simulink model "boat_dynamics_model"  (R2025a)
settings: Solver=ode4  StartTime=0.0  StopTime=10  FixedStep=Ts_sim  RelTol=1e-3
values from neighbouring files (symbols this model uses):
  ctrl_params = boat_controller_parameters()    [setup_MDL.m]
  plant_params = boat_model_parameters_3dof()    [setup_MDL.m]
  u0 = u0(:)    [find_A_B_LQR.m]    (also in find_equilibrium_3dof.m = zeros(5,1); setup_MDL.m = trim.u0; tmp_continuous_controller.mat = [1.84671066471 1.84671066471 1.93397466068 0 3]; tmp_discrete_controller.mat = [1.84671066471 1.84671066471 1.93397466068 0 3])
  x0 = x0(:)    [find_A_B_LQR.m]    (also in find_equilibrium_3dof.m = zeros(11,1); setup_MDL.m = trim.x0; tmp_continuous_controller.mat = [-0.1 0 0 0 0 0 0 0 1.84671066471 1.84671066471 1.9339746606; tmp_discrete_controller.mat = [-0.1 0 0 0 0 0 0 0 1.84671066471 1.84671066471 1.9339746606)
undefined symbols (not defined in the file or in its folder): Ts_sim
libraries: simulink_extras x2, sim3dlib x2, rllib x1
settings Model: Creator=brzan  LastModifiedBy=brzan

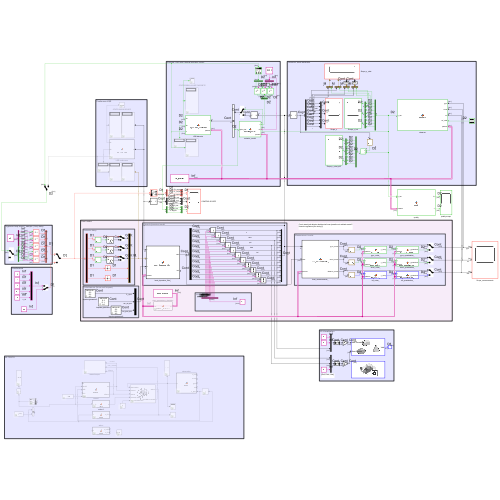
[thumbnail: Simulink's stored preview of the top-level diagram]
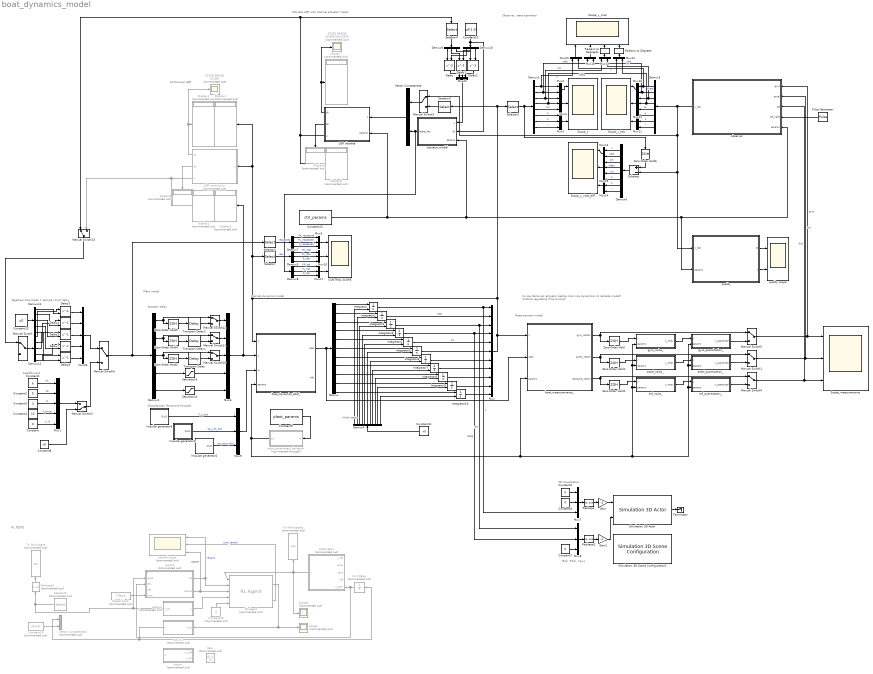
== system boat_dynamics_model ==
  note: Plant model
  note: Actuator delay
  note: Algebraic loop break 1 sample (1ms) delay
  note: RL TESTS
  note: Observer, state estimator
  note: Co sie stanie jak aktuator bedzie mial inna dynamike niz zaklada model?
      | Uczenie regulatora (fine tuning?)
  note: Discrete LQR with Internal actuator model
  note: Continuous LQR
  note: Feedforward
  note: Measurement model
  note: Internal dynamics model
  note: Initial state
  note: Disturbances (force and forques)
  note: 3D Visualization
  note: [Roll, Pitch, Yaw]
  CONTROL SCOPE : Scope  NumInputPorts=3
      settings: ActiveDisplayYMinimum=1.6100937743534502  ActiveDisplayYMaximum=2.3589425832417694  DataLoggingVariableName=ScopeAction
  Constant{,5..7} (4 alike) : Constant  Value=0
  Constant1 : Constant  Value=6
  Constant10 : Constant  Value=u0(1:3)  VectorParams1D=off
  Constant11 : Constant  Value=x0  VectorParams1D=off
  Constant12 : Constant  Value=u0  VectorParams1D=off
  Constant13 : Constant  Value=ctrl_params  VectorParams1D=off  OutDataTypeStr=Bus: ctrl_params_bus
  Constant14 : Constant  Commented=on  Value=u0(4:5)  VectorParams1D=off
  Constant15 : Constant  Commented=on  Value=0
  Constant2 : Constant  Value=6
  Constant3 : Constant  Value=3
  Constant4 : Constant  Value=10
  Constant8 : Constant  Value=u0
  Constant9 : Constant  Value=plant_params  VectorParams1D=off  OutDataTypeStr=Bus: plant_params_bus
  Delay : Delay  DelayLength=3  InitialConditionSource=Input port  SampleTime=ctrl_params.Ts
      settings: InputPortMap=u0,p4
  Delay1 : Delay  DelayLength=3  InitialConditionSource=Input port  SampleTime=ctrl_params.Ts
      settings: InputPortMap=u0,p4
  Delay2 : Delay  DelayLength=3  InitialConditionSource=Input port  SampleTime=ctrl_params.Ts
      settings: InputPortMap=u0,p4
  Delay{3..5,7..8} (5 alike) : Delay  DelayLength=1  InitialConditionSource=Input port  SampleTime=Ts_sim
      settings: InputPortMap=u0,p4
  Demux : Demux  Outputs=11
  Demux1 : Demux  Outputs=8
  Demux{3,7..10} (5 alike) : Demux  Outputs=3
  Demux11 : Demux  Outputs=5
  Demux12 : Demux  Outputs=5
  Demux2 : Demux  Outputs=5
  Demux4 : Demux  Outputs=11
  Demux5 : Demux  Outputs=8
  Demux6 : Demux  Outputs=8
  Digital Clock : DigitalClock  Commented=on  SampleTime=0.01
  Display{1..8} (8 alike) : Display  Commented=on
  Gain : Gain  Gain=-1
  Gain1 : Gain  Gain=-1
  Impulse generator1 : Subsystem  mask{start=2, duration=.1, amplitude=0}
      mask prompts: start "Start time"; duration "Duration time"; amplitude "Impulse amplitude"
      mask Display:
      | disp([ ...
      |     "IMPULSE"; ...
      |     'S ', ...
      |     num2str(get_param(gcb, 'start')); ...
      |     'D ', ...
      |     num2str(get_param(gcb, "duration")); ...
      |     'A ', ...
      |     num2str(get_param(gcb, "amplitude")) ...
      | ]);
  Impulse generator2 : Subsystem  mask{start=2, duration=5, amplitude=0}
      mask prompts: start "Start time"; duration "Duration time"; amplitude "Impulse amplitude"
      mask Display:
      | disp([ ...
      |     "IMPULSE"; ...
      |     'S ', ...
      |     num2str(get_param(gcb, 'start')); ...
      |     'D ', ...
      |     num2str(get_param(gcb, "duration")); ...
      |     'A ', ...
      |     num2str(get_param(gcb, "amplitude")) ...
      | ]);
  Impulse generator3 : Subsystem  mask{start=0, duration=2, amplitude=0}
      mask prompts: start "Start time"; duration "Duration time"; amplitude "Impulse amplitude"
      mask Display:
      | disp([ ...
      |     "IMPULSE"; ...
      |     'S ', ...
      |     num2str(get_param(gcb, 'start')); ...
      |     'D ', ...
      |     num2str(get_param(gcb, "duration")); ...
      |     'A ', ...
      |     num2str(get_param(gcb, "amplitude")) ...
      | ]);
  Integrator : Integrator  InitialConditionSource=external  InitialCondition=-0.11
  Integrator{1,3..10} (9 alike) : Integrator  InitialConditionSource=external
  Integrator2 : Integrator  InitialConditionSource=external  InitialCondition=deg2rad(3)
  LQR continuous : MATLAB Function  Commented=on  TreatAsAtomicUnit=on
  LQR discrete : MATLAB Function  TreatAsAtomicUnit=on  SystemSampleTime=ctrl_params.Ts
  Manual Switch{,1,3..6,10..13} (10 alike) : ManualSwitch
  Manual Switch2 : ManualSwitch  CurrentSetting=0
  Mux : Mux  Inputs=11
  Mux1 : Mux  Inputs=5
  Mux{2,10,13,18..21} (7 alike) : Mux  Inputs=2
  Mux{3..5,7..9,11..12,14..17,22} (13 alike) : Mux  Inputs=3
  Mux23 : Mux  Inputs=5
  Mux6 : Mux  Inputs=5
  Pulse Generator : DiscretePulseGenerator  Period=10  SampleTime=ctrl_params.Ts
  RL Agent : rllib/RL Agent  Commented=on  Agent=agentObj  ExternalActionAsInput=on  ProvideLastAction=off  ProvideCumRwd=on  TreatAsDirectFeedthrough=on  UseStrictObservationDataTypes=off
  Radians to Degrees : simulink_extras/Transformations/Radians to Degrees
  Radians to Degrees1 : simulink_extras/Transformations/Radians to Degrees
  Reshape : Reshape  OutputDimensionality=Row vector (2-D)
  Reshape1 : Reshape  OutputDimensionality=Row vector (2-D)
  Reshape2 : Reshape  Commented=on
  STATE ERROR SCOPE : Scope  Commented=on
      settings: ActiveDisplayYMinimum=-0.17004569092279864  ActiveDisplayYMaximum=0.25579071640803624  DataLoggingVariableName=ScopeData3
  STATE ERROR SCOPE DISCRETE : Scope  Commented=on
      settings: ActiveDisplayYMinimum=-0.17004569092279864  ActiveDisplayYMaximum=0.25579071640803624  DataLoggingVariableName=ScopeData6
  Saturation3 : Saturate  UpperLimit=5  LowerLimit=0
  Saturation4 : Saturate  UpperLimit=5  LowerLimit=0
  Scope : Scope  Commented=on
      settings: ActiveDisplayYMinimum=-2.4199088465030929  ActiveDisplayYMaximum=1.3794615097714347  DataLoggingVariableName=ScopeData2
  Scope1 : Scope  Commented=on
      settings: ActiveDisplayYMinimum=0.99404961030066707  ActiveDisplayYMaximum=1.0007752200523612  DataLoggingVariableName=ScopeData4
  Scope_measurements : Scope  NumInputPorts=3
      settings: ActiveDisplayYMinimum=-1.41006075  ActiveDisplayYMaximum=1.1051827499999998
  Scope_x : Scope  NumInputPorts=3
      settings: ActiveDisplayYMinimum=-0.11336426588314241  ActiveDisplayYMaximum=0.018631710839364757
  Scope_x_hat : Scope  NumInputPorts=3
      settings: ActiveDisplayYMinimum=-0.16104234357264974  ActiveDisplayYMaximum=0.14683807575538765  DataLoggingVariableName=ScopeObservation
  Scope_x_xhat : Scope  NumInputPorts=4
      settings: ActiveDisplayYMinimum=-0.24045599939750117  ActiveDisplayYMaximum=0.052378489407279127  DataLoggingVariableName=ScopeData7
  Scope_x_xhat_diff : Scope  NumInputPorts=3
      settings: ActiveDisplayYMinimum=-0.10989376677955481  ActiveDisplayYMaximum=0.074956658726200817  DataLoggingVariableName=ScopeData5
  Selector : Selector  InputPortWidth=11  IndexOptions=Index vector (dialog)  Indices=[9 10 11]  OutputSizes=1
  Selector1 : Selector  InputPortWidth=5  IndexOptions=Index vector (dialog)  Indices=[1 2 3]  OutputSizes=1
  Selector2 : Selector  InputPortWidth=11  IndexOptions=Index vector (dialog)  Indices=[1 2 3 4 5 6 7 8]  OutputSizes=1
  Selector3 : Selector  InputPortWidth=11  IndexOptions=Index vector (dialog)  Indices=[1 2 3 4 5 6 7 8]  OutputSizes=1
  Selector4 : Selector  InputPortWidth=5  IndexOptions=Index vector (dialog)  Indices=[1 2 3]  OutputSizes=1
  Selector5 : Selector  Commented=on  InputPortWidth=5  IndexOptions=Index vector (dialog)  Indices=[1 2 3]  OutputSizes=1
  Simulation 3D Actor : sim3dlib/Simulation 3D Actor  Priority=1  ActorName=Boat  ParentName=Scene Origin  Operation=Create at setup  InitScriptText=|  SampleTime=-1  Translation=[0 0 0]  Rotation=[0 0 0]  Scale=[1 1 1]/1000  InputsText=Boat.Translation Boat.Rotation  aMode=5  ActorTag=Boat  ActorType=Sim3dActor  ID=C
      | % Reserved keywords:
      | % - Actor : handle to this actor object
      | % - World : handle to the world object
      | 
      | % Examples:
      | 
      | % Create a primitive geometry (optional)
      | % createShape(Actor, 'box', [1 1 1]);
      | 
      | % Initialize values (optional)
      | % Actor.Physics = true;
      | % Actor.Color = [1 0 0];
  Simulation 3D Scene Configuration1 : sim3dlib/Simulation 3D Scene Configuration  Priority=0  ProjectFormat=Default Scenes  SceneDesc=Open surface  ProjectName=C:\Program Files\MATLAB\R2025a\toolbox\shared\sim3d_projects\automotive_project_windows\UE\WindowsNoEditor\VehicleSimulation.exe  ScenePath=/Game/Maps/HwStrght  EnableOpenDRIVE=off  vehTagList={'Boat';'Custom';'Scene Origin'}  vehTag=Boat  AttachedCameraRelativeTranslation=[-4 -3 1]*1000*0.25  FreeCameraDefaultInitialTranslation=[-6, 0, 2]  AttachedCameraRelativeRotation=[0 -10 40]  FreeCameraDefaultInitialRotation=[0, -15, 0]  ViewpointName=Custom  FreeCameraInitialTranslation=[-5 0 1]  ViewpointTranslation=[0 0 0]  FreeCameraInitialRotation=[0 0 0]  ViewpointRotation=[0 0 0]  OpVisEn=off  Ts=.05  EnableWindow=on  EnableRemoteAccess=off  EnableWeather=off  SunAzimuth=90  SunAltitude=40.0  EnableGeospatialSun=off  Latitude=0  Longitude=0  Date=2023-01-01  Time=10:30:00  GeoTimeZone=-5.0  SunDaylightSaving=off  wind=1  clouds=10  EnableVolumetricClouds=off  CloudCoverage=0  CloudAltitude=6  fog=0  rain=0  RaindropsEffect=off  SnowDensity=0  EnableGeospatial=off  TilesetSource=Earth terrain  UseTrueOrigin=off  OriginHeight=200  OriginLatitude=40.744652  OriginLongitude=-73.988864  MapStyle=Aerial  AdditionalAssetIDs=[]  UseAdvancedSunSky=off  SolarTime=11  TimeZone=-5  Day=21  Month=9  Year=2022  UseDaylightSavingTime=on  DSTStartDay=10  DSTStartMonth=3  DSTEndDay=3  DSTEndMonth=11  DSTSwitchHour=2  sensorTag=MainCamera1  sensorId=1  sensorName=MainCamera1  mountLoc=Origin  offsetFlag=off  tmountOffset=[0, 0, 0]  rmountOffset=[0, 0, 0]  HorizontalResolution=1280  VerticalResolution=720  HorizontalFOV=60  mountPoint=[0 0 0]  mountOrientation=[0 0 0]  aMode=5  ID=1  GeoTrigger=Inactive  ViewNameList={'Custom'}  ViewTranslationList={'[-5 0 1]'}  ViewRotationList={'[0 0 0]'}
      settings: LibrarySourceBlock=sl3dlib/Simulation 3D/Environment/Simulation 3D Scene Configuration
  Subtract : Sum  Inputs=+-
  Terminator : Terminator
  To Workspace : ToWorkspace  Commented=on  VariableName=act  SaveFormat=Structure With Time  SampleTime=-1
  To Workspace1 : ToWorkspace  Commented=on  VariableName=obs  SaveFormat=Structure With Time  SampleTime=-1
  Transport Delay : TransportDelay  DelayTime=plant_params.hydrofoils.dynamics.L  InitialOutput=u0(3)
  Transport Delay1 : TransportDelay  DelayTime=plant_params.hydrofoils.dynamics.L  InitialOutput=u0(2)
  Transport Delay2 : TransportDelay  DelayTime=plant_params.hydrofoils.dynamics.L  InitialOutput=u0(1)
  Unit Delay : UnitDelay  Commented=on  InitialCondition=u0(1:3)  SampleTime=0.01  HasFrameUpgradeWarning=on
  Vector Concatenate : Concatenate
  Vector Concatenate1 : Concatenate  Commented=on
  Zero : Constant  Commented=on  Value=[0; 0; 0]  OutDataTypeStr=Inherit: Inherit via back propagation
  Zero-Order Hold : ZeroOrderHold  SampleTime=plant_params.gyro.sample_time
  Zero-Order Hold1 : ZeroOrderHold  SampleTime=plant_params.accel.sample_time
  Zero-Order Hold2 : ZeroOrderHold  SampleTime=plant_params.tof.sample_time
  Zero-Order Hold3 : ZeroOrderHold  SampleTime=plant_params.hydrofoils.dynamics.Ts_act
  Zero-Order Hold4 : ZeroOrderHold  SampleTime=plant_params.hydrofoils.dynamics.Ts_act
  Zero-Order Hold5 : ZeroOrderHold  SampleTime=plant_params.hydrofoils.dynamics.Ts_act
  Zero-Order Hold6 : ZeroOrderHold  SampleTime=ctrl_params.Ts
  accel_noise_ : MATLAB Function  TreatAsAtomicUnit=on  SystemSampleTime=plant_params.accel.sample_time
  accel_quantization_ : MATLAB Function  TreatAsAtomicUnit=on  SystemSampleTime=plant_params.accel.sample_time
  action : MATLAB Function  Commented=on  TreatAsAtomicUnit=on
  action1 : MATLAB Function  Commented=on  TreatAsAtomicUnit=on
  action2 : MATLAB Function  Commented=on  TreatAsAtomicUnit=on
  actuator_model : MATLAB Function  TreatAsAtomicUnit=on  SystemSampleTime=ctrl_params.Ts
  boat_dynamics_3dof_ : MATLAB Function  TreatAsAtomicUnit=on
  boat_measurements_ : MATLAB Function  TreatAsAtomicUnit=on
  gyro_noise_ : MATLAB Function  TreatAsAtomicUnit=on  SystemSampleTime=plant_params.gyro.sample_time
  gyro_quantization_ : MATLAB Function  TreatAsAtomicUnit=on  SystemSampleTime=plant_params.gyro.sample_time
  observation : MATLAB Function  Commented=on  TreatAsAtomicUnit=on  SystemSampleTime=0.01
  observer : MATLAB Function  TreatAsAtomicUnit=on  SystemSampleTime=ctrl_params.Ts
  plant_parameters_deviation : MATLAB Function  Commented=through  TreatAsAtomicUnit=on
  quality : MATLAB Function  TreatAsAtomicUnit=on  SystemSampleTime=ctrl_params.Ts
  quality scope : Scope  NumInputPorts=2
      settings: ActiveDisplayYMinimum=-0.12455482970730834  ActiveDisplayYMaximum=1.1240659773755071  DataLoggingVariableName=ScopeData8
  reward : MATLAB Function  Commented=on  TreatAsAtomicUnit=on  SystemSampleTime=ctrl_params.Ts
  reward scope : Scope  Commented=on  NumInputPorts=3
      settings: ActiveDisplayYMinimum=-2399.5814447480943  ActiveDisplayYMaximum=277.10834326270424  DataLoggingVariableName=ScopeData9
  tof_noise_ : MATLAB Function  TreatAsAtomicUnit=on  SystemSampleTime=plant_params.tof.sample_time
  tof_quantization_ : MATLAB Function  TreatAsAtomicUnit=on  SystemSampleTime=plant_params.tof.sample_time
  wires:
  boat_dynamics_3dof_/1(xdot) -> boat_measurements_/2(xdot), Demux/1
  Constant9/1 -> plant_parameters_deviation/1(in)
  Demux/1 -> Integrator/1
  Demux/2 -> Integrator1/1
  Demux/4 -> Integrator3/1
  Demux/3 -> Integrator2/1
  Demux/5 -> Integrator4/1
  Demux/6 -> Integrator5/1
  Integrator/1 -> Mux7/3, Mux/1  "z"
  Integrator1/1 -> Mux/2  "zdot"
  Integrator2/1 -> Mux/3, Mux8/1  "phi"
  Integrator3/1 -> Mux/4, Mux8/2  "theta"
  Integrator4/1 -> Mux/5  "ksi"
  Integrator5/1 -> Mux/6
  Constant/1 -> Mux1/5  "V_W"
  Constant1/1 -> Mux1/1  "FL"
  Constant4/1 -> Mux1/4  "F_thrust"
  Demux1/1 -> Mux20/1, Mux2/1  "z"
  Mux2/1 -> Scope_x/1
  Demux1/2 -> Mux2/2, Mux18/1  "zdot"
  Constant3/1 -> Mux1/3  "R"
  Constant2/1 -> Mux1/2  "FR"
  Constant5/1 -> Mux7/1
  Constant6/1 -> Mux7/2
  Mux8/1 -> Reshape1/1
  Mux7/1 -> Reshape/1
  Reshape/1 -> Gain/1
  Simulation 3D Actor/1 -> Terminator/1
  Gain1/1 -> Simulation 3D Actor/2
  Reshape1/1 -> Gain1/1
  Constant7/1 -> Mux8/3
  Demux/7 -> Integrator6/1
  Demux/8 -> Integrator7/1
  Integrator6/1 -> Mux/7
  Integrator7/1 -> Mux/8
  Demux1/3 -> Mux19/1, Mux4/1  "phi"
  Demux1/4 -> Mux21/1, Mux4/2  "theta"
  Demux1/5 -> Mux4/3  "ksi"
  Demux1/6 -> Mux3/1  "p"
  Demux1/7 -> Mux3/2  "q"
  Demux1/8 -> Mux3/3  "r"
  Mux4/1 -> Scope_x/2
  Mux3/1 -> Scope_x/3
  Manual Switch1/1 -> observer/2(accel), Scope_measurements/2  "acc"
  Manual Switch4/1 -> observer/3(tof), Scope_measurements/3  "dist"
  gyro_noise_/1(y_noisy) -> gyro_quantization_/1(y)
  Zero-Order Hold/1 -> gyro_noise_/1(y)
  boat_measurements_/1(gyro_vector) -> Manual Switch5/1, Zero-Order Hold/1
  Manual Switch5/1 -> Scope_measurements/1, observer/1(gyro)  "gyro"
  gyro_quantization_/1(y_quantized) -> Manual Switch5/2
  boat_measurements_/3(distance_vector) -> Zero-Order Hold2/1, Manual Switch4/1
  boat_measurements_/2(accel_vector) -> Manual Switch1/1, Zero-Order Hold1/1
  Zero-Order Hold2/1 -> tof_noise_/1(y)
  Zero-Order Hold1/1 -> accel_noise_/1(y)
  accel_noise_/1(y_noisy) -> accel_quantization_/1(y)
  tof_noise_/1(y_noisy) -> tof_quantization_/1(y)
  accel_quantization_/1(y_quantized) -> Manual Switch1/2
  LQR continuous/3(u) -> Manual Switch13/2, Display2/1
  LQR continuous/2(du) -> Display5/1
  LQR continuous/1(dx) -> STATE ERROR SCOPE/1, Display1/1
  plant_parameters_deviation/1(out) -> boat_measurements_/3(params), tof_noise_/2(params), accel_noise_/2(params), gyro_noise_/2(params), gyro_quantization_/2(params), accel_quantization_/2(params), tof_quantization_/2(params), boat_dynamics_3dof_/4(params)
  Saturation3/1 -> Mux6/4
  Saturation4/1 -> Mux6/5
  Manual Switch6/1 -> Selector1/1, Demux2/1
  Demux2/4 -> Saturation3/1
  Demux2/5 -> Saturation4/1
  Demux2/3 -> Zero-Order Hold3/1, Manual Switch10/1
  Transport Delay/1 -> Manual Switch10/2
  Demux2/2 -> Zero-Order Hold4/1, Manual Switch11/1
  Transport Delay1/1 -> Manual Switch11/2
  Demux2/1 -> Manual Switch12/1, Zero-Order Hold5/1
  Transport Delay2/1 -> Manual Switch12/2
  Manual Switch10/1 -> Mux6/3
  Manual Switch11/1 -> Mux6/2
  Manual Switch12/1 -> Mux6/1
  Gain/1 -> Simulation 3D Actor/1
  Mux9/1 -> boat_dynamics_3dof_/3(w)
  Impulse generator3/1(Out1) -> Mux9/1  "F_z_dist"
  Impulse generator1/1(Out1) -> Mux9/2  "tau_roll_dist"
  Impulse generator2/1(Out1) -> Mux9/3  "tau_pitch_dist"
  Demux4/1 -> Integrator/2
  Demux4/8 -> Integrator7/2
  Demux4/2 -> Integrator1/2
  Demux4/3 -> Integrator2/2
  Demux4/4 -> Integrator3/2
  Demux4/5 -> Integrator4/2
  Demux4/6 -> Integrator5/2
  Demux4/7 -> Integrator6/2
  Constant11/1 -> Demux4/1
  Mux10/1 -> Scope_x_hat/1
  Mux12/1 -> Scope_x_hat/2
  Mux11/1 -> Scope_x_hat/3
  Demux5/8 -> Mux11/3  "r"
  Demux5/7 -> Mux11/2  "q"
  Demux5/6 -> Mux11/1  "p"
  Demux5/5 -> Mux12/3  "ksi"
  Demux5/4 -> Mux21/2, Mux12/2  "theta"
  Demux5/3 -> Mux19/2, Mux12/1  "phi"
  Demux5/2 -> Mux18/2, Mux10/2  "zdot"
  Demux5/1 -> Mux20/2, Mux10/1  "z"
  Pulse Generator/1 -> observer/4(tof_valid)
  Demux6/8 -> Mux14/3  "r"
  Demux6/2 -> Mux13/2  "zdot"
  Demux6/3 -> Mux15/1  "phi"
  Mux13/1 -> Scope_x_xhat_diff/1
  Demux6/1 -> Mux13/1  "z"
  Mux15/1 -> Scope_x_xhat_diff/2
  Mux14/1 -> Scope_x_xhat_diff/3
  Demux6/5 -> Mux15/3  "ksi"
  Subtract/1 -> Demux6/1
  Demux6/4 -> Mux15/2  "theta"
  Demux6/7 -> Mux14/2  "q"
  Demux6/6 -> Mux14/1  "p"
  LQR discrete/2(du) -> Display6/1
  LQR discrete/1(dx) -> STATE ERROR SCOPE DISCRETE/1, Display7/1
  Mux/1 -> Selector/1, LQR continuous/1(x), Display4/1, boat_dynamics_3dof_/1(x), Selector3/1, Selector2/1, boat_measurements_/1(x)
  Manual Switch13/1 -> Manual Switch/1
  Mux23/1 -> Manual Switch6/1
  Demux/9 -> Integrator8/1
  Integrator8/1 -> Mux/9
  Integrator9/1 -> Mux/10
  Demux/10 -> Integrator9/1
  Integrator10/1 -> Mux/11
  Demux/11 -> Integrator10/1
  Demux4/9 -> Integrator8/2
  Demux4/10 -> Integrator9/2
  Demux4/11 -> Integrator10/2
  tof_quantization_/1(y_quantized) -> Manual Switch4/2
  Demux7/2 -> Mux5/2  "FL_requested"
  Demux7/3 -> Mux5/3  "R_requested"
  Mux5/1 -> CONTROL SCOPE/1
  Demux7/1 -> Mux5/1  "FR_requested"
  Selector1/1 -> Demux7/1  "requested"
  Demux3/1 -> Mux16/1  "FR_real"
  Selector/1 -> Demux3/1  "real"
  Mux16/1 -> CONTROL SCOPE/2
  Demux3/3 -> Mux16/3  "R_real"
  Demux3/2 -> Mux16/2  "FL_real"
  Mux6/1 -> Display3/1, boat_dynamics_3dof_/2(u)
  Constant8/1 -> Manual Switch2/2
  Mux1/1 -> Manual Switch2/1
  Selector2/1 -> Zero-Order Hold6/1, Demux1/1
  Zero-Order Hold4/1 -> Transport Delay1/1
  Zero-Order Hold5/1 -> Transport Delay2/1
  Zero-Order Hold3/1 -> Transport Delay/1
  actuator_model/1(alpha_hat) -> Demux8/1, Vector Concatenate/2
  Selector3/1 -> Manual Switch3/2
  Vector Concatenate/1 -> LQR discrete/1(x)
  Selector4/1 -> Demux9/1
  Demux8/1 -> Mux17/1  "FR_hat"
  Demux8/2 -> Mux17/2  "FL_hat"
  Mux17/1 -> CONTROL SCOPE/3
  Demux8/3 -> Mux17/3  "R_hat"
  Mux22/1 -> actuator_model/1(u)
  Manual Switch3/1 -> Vector Concatenate/1
  Zero-Order Hold6/1 -> Subtract/1
  Mux19/1 -> Radians to Degrees1/1
  Mux18/1 -> Scope_x_xhat/2
  Mux20/1 -> Scope_x_xhat/1
  Mux21/1 -> Radians to Degrees/1
  Constant10/1 -> actuator_model/2(u0), Demux10/1
  Demux9/1 -> Delay/1
  Demux9/2 -> Delay1/1
  Demux9/3 -> Delay2/1
  Demux10/1 -> Delay/2
  Demux10/2 -> Delay1/2
  Demux10/3 -> Delay2/2
  Delay1/1 -> Mux22/2
  Delay/1 -> Mux22/1
  Delay2/1 -> Mux22/3
  Demux11/1 -> Delay3/2
  Demux12/3 -> Delay5/1
  Delay3/1 -> Mux23/1
  Demux11/2 -> Delay4/2
  Demux12/2 -> Delay4/1
  Demux12/1 -> Delay3/1
  Delay4/1 -> Mux23/2
  Demux11/3 -> Delay5/2
  Constant12/1 -> Demux11/1
  Constant13/1 -> LQR discrete/2(params), actuator_model/3(params), observer/5(params), quality/2(params)
  quality/1(Q) -> quality scope/1
  quality/2(J) -> quality scope/2
  reward/2(isDone) -> reward scope/3, RL Agent/3  "isDone"
  reward/1(ret) -> RL Agent/2, reward scope/1  "reward"
  observer/1(x_hat) -> Subtract/2, quality/1(x_hat), Manual Switch3/1, Demux5/1
  Manual Switch2/1 -> Manual Switch6/2
  Constant14/1 -> Vector Concatenate1/2
  Manual Switch/1 -> Demux12/1
  Radians to Degrees/1 -> Scope_x_xhat/4
  Radians to Degrees1/1 -> Scope_x_xhat/3
  LQR discrete/3(u) -> Manual Switch13/1, Selector4/1, Display8/1
  Selector5/1 -> reward/2(uLQR), action2/1(u_RL), Reshape2/1
  RL Agent/2 -> reward scope/2  "cum_reward"
  Constant15/1 -> RL Agent/5
  Delay5/1 -> Mux23/3
  Demux11/4 -> Delay7/2
  Demux11/5 -> Delay8/2
  Demux12/4 -> Delay7/1
  Demux12/5 -> Delay8/1
  Delay8/1 -> Mux23/5
  Delay7/1 -> Mux23/4
  Reshape2/1 -> To Workspace/1
  Unit Delay/1 -> reward/3(uRL), observation/5(u_prev)
  observation/1(o) -> Scope1/1, To Workspace1/1, RL Agent/1
  RL Agent/1 -> Scope/1, action1/1(u_RL)
  Digital Clock/1 -> reward/5(time)
  action2/1(u) -> RL Agent/4
  action1/1(u) -> Unit Delay/1, Vector Concatenate1/1

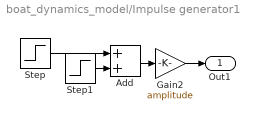
== system boat_dynamics_model/Impulse generator1 ==
  Add : Sum
  Gain2 : Gain  Gain=amplitude
  Step : Step  Time=start  SampleTime=0
  Step1 : Step  Time=start+duration  After=-1  SampleTime=0
  Out1 : Outport
  wires:
  Step/1 -> Add/1
  Step1/1 -> Add/2
  Gain2/1 -> Out1/1
  Add/1 -> Gain2/1

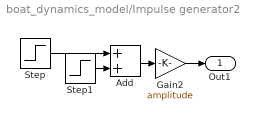
== system boat_dynamics_model/Impulse generator2 ==
  Add : Sum
  Gain2 : Gain  Gain=amplitude
  Step : Step  Time=start  SampleTime=0
  Step1 : Step  Time=start+duration  After=-1  SampleTime=0
  Out1 : Outport
  wires:
  Step/1 -> Add/1
  Step1/1 -> Add/2
  Gain2/1 -> Out1/1
  Add/1 -> Gain2/1

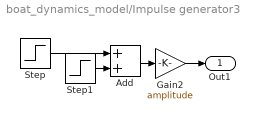
== system boat_dynamics_model/Impulse generator3 ==
  Add : Sum
  Gain2 : Gain  Gain=amplitude
  Step : Step  Time=start  SampleTime=0
  Step1 : Step  Time=start+duration  After=-1  SampleTime=0
  Out1 : Outport
  wires:
  Step/1 -> Add/1
  Step1/1 -> Add/2
  Gain2/1 -> Out1/1
  Add/1 -> Gain2/1

== matlab function boat_dynamics_model/plant_parameters_deviation ==
  data: in input Bus: plant_params_bus; out output Bus: plant_params_bus
function out = params_deviation(in) %#codegen
    out = in;

    % Introduce some variance
    % out.m = in.m * .8;
    % 
    % out.Ix_B = in.Ix_B * 1.2;
    % out.Iy_B = in.Iy_B * .8;
    % 
    % out.hydrofoils.dynamics.T = in.hydrofoils.dynamics.T * 1.2;
end

== matlab function boat_dynamics_model/observer ==
  data: gyro input; x_hat output size=8; accel input; tof input; tof_valid input; params input Bus: ctrl_params_bus
function x_hat = observer(gyro, accel, tof, tof_valid, params) %#codegen
% OBSERVER
% Estimates attitude (Mahony) and heave states (KF).
%
% Frames:
%   - World: NED (Z+ down)
%   - Body:  IMU / vehicle frame
%
% Inputs:
%   gyro      [3x1] deg/s   body angular rates                      [gx gy gz]
%   accel     [3x1] g       body acceleration (includes gravity)    [ax ay az]
%   tof       [4x1] mm      ToF distances to water                  [front_left, front_right, rear_left, rear_right]
%   tof_valid logical      new ToF available
%   params                controller/observer parameters
%
% Output:
%   x_hat = [
%       z;        % heave position [m]
%       z_dot;    % heave velocity [m/s]
%       phi;      % roll  [rad]
%       theta;    % pitch [rad]
%       psi;      % yaw   [rad] (unused)
%       p;        % roll rate  [rad/s]
%       q;        % pitch rate [rad/s]
%       r         % yaw rate   [rad/s] (unused)
%   ];
    %% Parameters

    Ts = params.Ts; % Block's sample time
    g = params.g; % gravity [m/s^2]

    %% Mahony attitude estimation
    persistent quat gyro_bias
    if isempty(quat) || isempty(gyro_bias)
        % quat = [1; 0; 0; 0];  % [qw qx qy qz], body->world
        gyro_bias = [0; 0; 0];     % gyro bias [rad/s]


        % accel is in g, body frame, NED (+Z down)
        a = accel / norm(accel);
    
        phi0   = atan2( a(2), a(3) );
        theta0 = atan2(-a(1), sqrt(a(2)^2 + a(3)^2));
        psi0   = 0; % yaw unobservable
    
        quat = eul2quat([psi0 theta0 phi0])'; % ZYX
    end

    [quat, gyro_bias, gyro_corr] = mahony_update(quat, gyro_bias, ...
                                                 deg2rad(gyro), accel, ...
                                                 params);

    [phi, theta, psi] = quat_to_euler_BW(quat);

    %% Heave Kalman Filter [z; z_dot; a_bias]
    persistent xh Pz
    if isempty(xh)
        z0 = tof_to_z(tof, phi, theta, params);
        xh = [z0; 0; 0];
        Pz = eye(3);
    end

    % compute vertical accel input a_z (m/s^2)
    aB = accel * g;
    aW = quat_rotate(quat, aB);
    a_z = aW(3) - g - xh(3);           % NED +down
    
    % KF predict with accel input and bias
    A = [1 Ts -0.5*Ts^2;
         0  1 -Ts;
         0  0  1];
    
    B = [0.5*Ts^2;
         Ts;
         0];
    
    % [z, z_dot, a_bias]
    Q = params.observer.heave_KF.Q;
    
    xh = A*xh + B*a_z;
    Pz = A*Pz*A' + Q;
    
    z      = xh(1);
    z_dot  = xh(2);
    % a_bias = xh(3);
    
    if tof_valid
        z_meas = tof_to_z(tof, phi, theta, params);
    
        H = [1 0 0];

        R = params.observer.heave_KF.R;
    
        % Update
        S = H*Pz*H' + R;
        K = Pz*H' / S;
        xh = xh + K*(z_meas - H*xh);
        Pz = (eye(3) - K*H)*Pz;
    
        z      = xh(1);
        z_dot  = xh(2);
        % a_bias = xh(3);
    end

    %% Output vector creation
    x_hat = [ ...
        z;
        z_dot;
        phi;
        theta;
        psi;          % psi yaw (unused)
        gyro_corr(1);
        gyro_corr(2);
        gyro_corr(3) % r yaw rate (unused)
    ];
end


function z = tof_to_z(tof, phi, theta, params)
% Convert ToF distances to heave position z (world, NED, meters)
%
% Inputs:
%   tof   [4x1]  distances in mm
%   phi           roll  [rad]
%   theta         pitch [rad]
%   params.tof.pos_*_B   sensor positions in BODY frame [m]
%
% Output:
%   z     scalar heave position [m], +down (NED)

    % Convert mm -> m
    d = tof * 1e-3;

    % Rotation (yaw irrelevant for vertical projection)
    cphi = cos(phi);   sphi = sin(phi);
    cth  = cos(theta); sth  = sin(theta);

    R_x = [1 0 0;
           0 cphi -sphi;
           0 sphi  cphi];

    R_y = [cth 0 sth;
           0   1 0;
          -sth 0 cth];

    R_BW = R_y * R_x;

    % ToF direction in world frame (body Z+ points down)
    e_B = [0; 0; 1];
    e_W = R_BW * e_B;

    ez = e_W(3);   % vertical projection

    % Sensor positions in world frame (relative to COM)
    rB = [ params.tof.pos_FL_B, ...
           params.tof.pos_FR_B, ...
           params.tof.pos_AL_B, ...
           params.tof.pos_AR_B ];

    rW = R_BW * rB;

    % Compute z estimate from each ToF
    z_i = -d .* ez - rW(3, :).';

    % Conservative fusion: average
    z = mean(z_i);
end

function [q, b, w] = mahony_update(q, b, gyro_rad_s, accel_g, params)

    % Gains 
    Kp = params.observer.attitude.Kp;
    Ki = params.observer.attitude.Ki;
    Ts = params.Ts;

    % Gate accel (gravity only)
    a_norm = norm(accel_g);
    use_acc = (a_norm > params.observer.attitude.acc_norm_min) && ...
              (a_norm < params.observer.attitude.acc_norm_max);

    if use_acc
        a = accel_g / a_norm;
        % Estimated gravity direction in BODY frame (NED: +Z down)
        g_est = quat_rotate(quat_conj(q), [0;0;1]);
        e = cross(a, g_est);
    else 
        e = [0;0;0];
    end

    % Bias update
    b = b + Ki * e * Ts;

    % Corrected gyro
    omega = gyro_rad_s - b + Kp * e;

    % Quaternion integration
    q_dot = 0.5 * quat_mul(q, [0; omega]);
    q = q + q_dot * Ts;
    q = q / norm(q);

    % Return correctec omega
    w = gyro_rad_s - b;
end


%% Smaller utility helpers
function qc = quat_conj(q)
    qc = [q(1); -q(2); -q(3); -q(4)];
end

function v = quat_rotate(q, v)
    v_q = quat_mul(quat_mul(q, [0; v]), quat_conj(q));
    v = v_q(2:4);
end

function q = quat_mul(a, b)
    q = [ ...
        a(1)*b(1) - a(2)*b(2) - a(3)*b(3) - a(4)*b(4);
        a(1)*b(2) + a(2)*b(1) + a(3)*b(4) - a(4)*b(3);
        a(1)*b(3) - a(2)*b(4) + a(3)*b(1) + a(4)*b(2);
        a(1)*b(4) + a(2)*b(3) - a(3)*b(2) + a(4)*b(1)];
end

function [phi, theta, psi] = quat_to_euler_BW(q)
    qw=q(1); qx=q(2); qy=q(3); qz=q(4);
    
    phi   = atan2(2*(qw*qx + qy*qz), 1 - 2*(qx^2 + qy^2));
    theta = asin( 2*(qw*qy - qz*qx));
    psi   = atan2(2*(qw*qz + qx*qy), 1 - 2*(qy^2 + qz^2));
end

== matlab function boat_dynamics_model/LQR discrete ==
  data: dx output; du output; x input; u output; params input
function [dx, du, u] = lqr_discrete_controller(x, params) %#codegen
    
    % Load once (persistent)
    persistent K u0 x0 ix iu
    if isempty(K)
        data = load('tmp_discrete_controller.mat');
        K  = data.Kd;
        u0 = data.u0;
        x0 = data.x0;
        ix = data.ix;
        iu = data.iu;
    end
    
    % State error
    dx = x - x0;
    
    % LQR control
    du = -K * dx(ix);
    
    % Full control input
    u = u0;
    u(1:3) = u0(1:3) + du;   % only flap commands
end

== matlab function boat_dynamics_model/actuator_model ==
  data: u input size=3; alpha_hat output size=3; u0 input; params input
function alpha_hat = actuator_model(u, u0, params) %#codegen
% Discrete actuator model (first-order lag)
%
% Inputs:
%   u_FL, u_FR, u_R   – commanded flap angles [deg]
%
% Outputs:
%   alpha_FL, alpha_FR, alpha_R – actual flap angles [deg]

    %% Persistent actuator states
    persistent alpha_FL_k alpha_FR_k alpha_R_k
    if isempty(alpha_FL_k)
        alpha_FL_k = u0(1);
        alpha_FR_k = u0(2);
        alpha_R_k  = u0(3);
    end

    %% Parameters from ctrl_params
    T  = params.actuator_model.T;   % actuator time constant [s]
    Ts = params.Ts;                 % controller sample time [s]

    alpha_min = params.actuator_model.alpha_min;   % [deg]
    alpha_max = params.actuator_model.alpha_max;   % [deg]

    %% Discrete coefficients ZOH
    a = exp(-Ts / T);
    b = 1.0 - a;

    %% Saturate commands
    u_FL = min(max(u(1), alpha_min), alpha_max);
    u_FR = min(max(u(2), alpha_min), alpha_max);
    u_R  = min(max(u(3),  alpha_min), alpha_max);

    %% Actuator dynamics update
    alpha_FL_k = a * alpha_FL_k + b * u_FL;
    alpha_FR_k = a * alpha_FR_k + b * u_FR;
    alpha_R_k  = a * alpha_R_k  + b * u_R;

    %% Outputs
    alpha_hat = [ alpha_FL_k; alpha_FR_k; alpha_R_k ];
end

== matlab function boat_dynamics_model/quality ==
  data: x_hat input; Q output; J output; params input
function [Q, J]  = quality(x_hat, params) %#codegen

    Ts  = params.Ts;
    tau = 1;   % 2–5 s
    alpha = Ts / tau;

    % Persistent state
    persistent J_avg
    if isempty(J_avg)
        J_avg = 0;
    end

    %% Unpack the x_hat
    z       = x_hat(1);      % [m]
    z_dot   = x_hat(2);      % [m/s]
    phi     = x_hat(3);      % [rad]
    theta   = x_hat(4);      % [rad]
    % ksi unused (5)
    p       = x_hat(6);      % [rad/s]
    q       = x_hat(7);      % [rad/s]
    % r unused (8)

    %% Reference
    z_ref       = -0.1;      % [m]
    z_dot_ref   = 0.0;       % [m/s]
    phi_ref     = 0.0;       % [rad]
    theta_ref   = 0.0;       % [rad]
    p_ref       = 0.0;       % [rad/s]
    q_ref       = 0.0;       % [rad/s]

    %% Scaling (acceptable errors)
    z_scal      = 0.08;         % [m]
    z_dot_scal  = 0.10;         % [m/s]
    phi_scal    = deg2rad(5);   % [rad]
    theta_scal  = deg2rad(5);   % [rad]
    p_scal      = deg2rad(20);  % [rad/s]
    q_scal      = deg2rad(20);  % [rad/s]

    %% Calculate the penalty 
    % J = weight * (error / scale)^2
    J_tot = ...
         1 * ((z     - z_ref)     / z_scal)     ^2 + ...
         1 * ((z_dot - z_dot_ref) / z_dot_scal) ^2 + ...
         1 * ((phi   - phi_ref)   / phi_scal)   ^2 + ...
         1 * ((theta - theta_ref) / theta_scal) ^2 + ...
         1 * ((p     - p_ref)     / p_scal)     ^2 + ...
         1 * ((q     - q_ref)     / q_scal)     ^2 + ...
         0;

    % TODO add more penalty for something like hull in water
    J_tot = J_tot + 0; 

    % 1st-order LPF on J
    J_avg = J_avg + alpha * (J_tot - J_avg);
   
    %% Calculate Quality
    J_inst = J_tot;
    J_long = J_avg;

    Q_inst = exp(-J_inst);
    Q_long = exp(-J_long);

    J = [J_inst, J_long];
    Q = [Q_inst, Q_long];

end

== matlab function boat_dynamics_model/reward ==
  data: x input; uLQR input; uRL input; info input; ret output; isDone output; time input
function [ret, isDone] = reward(x, uLQR, uRL, info, time) %#codegen
    ret = 0;
    isDone = false;
    % time

    %% Unpack the x state vector
    z       = x(1);     % [m]
    z_dot   = x(2);     % [m/s]
    phi     = x(3);     % [rad]
    theta   = x(4);     % [rad]
    ksi     = x(5);     % [rad] UNUSED
    p       = x(6);     % [rad/s]
    q       = x(7);     % [rad/s]
    r       = x(8);     % [rad/s] UNUSED
    % Actuator positions
    alpha_FL = x(9);    % [deg] 
    alpha_FR = x(10);   % [deg]
    alpha_R  = x(11);   % [deg]

    %% Unpack the u and compute the error
    eFL = uLQR(1) - uRL(1); % [deg]
    eFR = uLQR(2) - uRL(2);
    eR = uLQR(3) - uRL(3);

    %% Unpack the info state vector
    z_FL = info(1);     % [m]
    z_FR = info(2);     % [m]
    z_R  = info(3);     % [m]
    V_submerged = info(4); % [m^3]
    tau_roll  = info(5);   % [Nm]
    tau_pitch = info(6);   % [Nm]   
    tau_yaw   = info(7);   % [Nm] UNUSED
    V_W       = info(8);   % [m/s]

    %% Define the parameters such as 
    % Reference
    z_ref = -0.1; % [m]
    
    % Scaling
    z_scal = 0.04; % [m]
    phi_scal   = deg2rad(4);   % [rad]
    theta_scal = deg2rad(8);   % [rad]
    p_scal     = deg2rad(64);  % [rad/s]
    q_scal     = deg2rad(128);  % [rad/s]

    % LQR scalling
    alpha_scal = 2; % [deg]

    % etc
    % V_too_deep_threshold = 0.002; % [m^3] FIXME example value

    %% Compute helpful variables
    in_water_FL = z_FL > 0.002;  % in water if z is greater than -0.002 m threshold
    in_water_FR = z_FR > 0.002;  % -0.002 
    in_water_R  = z_R  > 0.002;

    % hull_too_deep = V_submerged > V_too_deep_threshold;

    %% Compute the reward

    % Height penalty
    % ret = ret - ((z - z_ref)/z_scal)^2;
    % Attitude penalty
    % ret = ret - (phi/phi_scal)^2 - (theta/theta_scal)^2;
    % Rate penalty (damping)
    % ret = ret - (p/p_scal)^2 - (q/q_scal)^2;

    % LQR imitation error penalty
    ret = ret - ( (eFL/alpha_scal)^2 + (eFR/alpha_scal)^2 + (eR/alpha_scal)^2 );

    % If any foil near surface of water - penalty
    if ~in_water_FL || ~in_water_FR || ~in_water_R
        % ret = ret - 10;
        % ret = ret - 1;
    end

    % % If hull deep in water - penalty
    % if hull_too_deep
    %     % ret = ret - 1000; TODO FIXME
    % end

    % Reward for being alive (typical controller run costs 6400 per 1000)
    ret = ret + 60;
    % ret = ret + 100;

    %% Episode termination
    isDone = termination(x, info);

    %% Termination penalty
    if isDone 
        ret = ret -  10000 + time * 100;

        if time < 0.8
            ret = ret - 1000;
        end
    end

end

function isDone = termination(x, info) %#codege
    
    phi   = x(3);
    theta = x(4);

    z_FL = info(1);     % [m]
    z_FR = info(2);     % [m]
    z_R  = info(3);     % [m]
    V_submerged = info(4);

    isDone = false;

    % If roll > 60 deg or pitch > 40 deg 
    if abs(phi) > deg2rad(60) || abs(theta) > deg2rad(40)
        isDone = true;
    end

    % If any foil out of water - termination
    in_water_FL = z_FL > 0.0;  % in water if z is greater than -0.0 m threshold
    in_water_FR = z_FR > 0.0; 
    in_water_R  = z_R  > 0.0;

    if ~in_water_FL || ~in_water_FR || ~in_water_R
        isDone = true;
    end
    
    % % If submerged ~ 60% of volume TODO FIXME
    % if V_submerged > 0.002
    %     % isDone = true;
    % end

end

== matlab function boat_dynamics_model/action ==
  data: u_LQR input; u output; u_RL input
function u = action(u_LQR, u_RL) %#codegen
    % Residual authority [deg]
    du_max = .5;

    % Residual in degrees
    du = clamp(u_RL, -1, 1) * du_max;

    % Additive residual control
    u = u_LQR + du;
end

function y = clamp(x, lb, ub)
    y = min(max(x, lb), ub);
end

== matlab function boat_dynamics_model/observation ==
  data: x_hat input; o output; accel input; gyro input; tof input; u_prev input
function o = observation(x_hat, accel, gyro, tof, u_prev) %#codegen
    
    z_ref = -0.1; % [m]

    %% Unpack and scale x_hat
    % z target is 0.1 i do not expect outside [0 -0.2] range but i would
    % prefer to keep the range broader a bit, by 0.1 in both directions
    % [0.1 -0.3] just in case...
    zen = clamp((x_hat(1) - z_ref) / 0.2, -1, 1);
    zdotn  = clamp(x_hat(2)/1, -1, 1); % [m/s] normalized by 

    phi   = x_hat(3);   % rad
    theta = x_hat(4);   % rad

    p_n     = clamp(x_hat(6) / deg2rad(100), -1, 1);   % rad/s normalized by 100 dps to [-1 1]
    q_n     = clamp(x_hat(7) / deg2rad(100), -1, 1);   % rad/s normalized by 100 dps to [-1 1]
    
    
    %% Unpack and scale accel
    % range is +/-2 [G]
    an = clamp(accel - [0; 0; 1] / 1.0, -1, 1); 

    %% Unpack and scale gyro
    % range is +/-2000 [dps] 
    % scaled_gyro = gyro / 2000;

    %% Unpack and scale tof
    % range is 0...255 [mm] 
    % scaled_tof = tof / 255; to 0-1 range
    % NOT USED, IT IS REDUNDANT idk?

    %% Unpack and scale control request
    % Control signal is in range -6/+12 [deg]
    % map [-6 .. +12] deg → [-1 .. +1]
    u_prev_n = (u_prev - 3.0) / 9.0;

    %% Build meaningful observation vector for the RL agent
    o = [
        zen;
        zdotn;
    
        sin(phi);
        cos(phi);
        sin(theta);
        cos(theta);
    
        p_n;
        q_n;
    
        % an(1);
        % an(2);
        an(3); % z component only xd
    
        u_prev_n(1);
        u_prev_n(2);
        u_prev_n(3)
    ];
end

function y = clamp(x, lb, ub)
    y = min(max(x, lb), ub);
end

== matlab function boat_dynamics_model/action1 ==
  data: u output; u_RL input
function u = action(u_RL) %#codegen
    u = (u_RL * 9) + 3;
end

% function y = clamp(x, lb, ub)
%     y = min(max(x, lb), ub);
% end

== matlab function boat_dynamics_model/action2 ==
  data: u output; u_RL input
function u = action(u_RL) %#codegen
    u = (u_RL - 3) / 9;
end

% function y = clamp(x, lb, ub)
%     y = min(max(x, lb), ub);
% end

== matlab function boat_dynamics_model/boat_dynamics_3dof_ ==
  data: x input; xdot output size=[11,1]; u input; w input; params input size=1; info output
function [ xdot, info ] = boat_dynamics_3dof_(x, u, w, params) %#codegen

    [ xdot, info ] = boat_dynamics_3dof(x, u, w, params);

end

== matlab function boat_dynamics_model/boat_measurements_ ==
  data: x input; xdot input; gyro_vector output; params input; accel_vector output; distance_vector output
function [ gyro_vector, accel_vector, distance_vector ] = boat_measurements_(x, xdot, params) %#codegen
    [ gyro_vector, accel_vector, distance_vector ] = boat_measurements(x, xdot, params);
end

== matlab function boat_dynamics_model/gyro_noise_ ==
  data: y input; y_noisy output; params input
function y_noisy = gyro_noise_(y, params) %#codegen
    % White noise
    y_noisy = y + params.gyro.noise_sigma .* randn(size(y));
end

== matlab function boat_dynamics_model/gyro_quantization_ ==
  data: y input; y_quantized output; params input
function y_quantized = gyro_quantization_(y, params) %#codegen
    y_quantized = params.gyro.quantization_step .* round(y ./ params.gyro.quantization_step);
end

== matlab function boat_dynamics_model/accel_noise_ ==
  data: y input; y_noisy output; params input
function y_noisy = accel_noise_(y, params) %#codegen
    % White noise
    y_noisy = y + params.accel.noise_sigma .* randn(size(y));
end

== matlab function boat_dynamics_model/tof_noise_ ==
  data: y input; y_noisy output; params input
function y_noisy = tof_noise_(y, params) %#codegen
    % White noise linearly dependant on distance
    sigma = params.tof.noise_sigma_a .* y + params.tof.noise_sigma_b;
    y_noisy = y + sigma .* randn(size(y));
end

== matlab function boat_dynamics_model/accel_quantization_ ==
  data: y input; y_quantized output; params input
function y_quantized = accel_quantization_(y, params) %#codegen
    y_quantized = params.accel.quantization_step .* round(y ./ params.accel.quantization_step);
end

== matlab function boat_dynamics_model/tof_quantization_ ==
  data: y input; y_quantized output; params input
function y_quantized = tof_quantization_(y, params) %#codegen
    y_quantized = params.tof.quantization_step .* round(y ./ params.tof.quantization_step);
end

== matlab function boat_dynamics_model/LQR continuous ==
  data: dx output; du output; x input; u output
function [dx, du, u] = lqr_controller(x) %#codegen

    % Load once (persistent)
    persistent K u0 x0 ix iu
    if isempty(K)
        data = load('tmp_continuous_controller.mat');
        % data = load('tmp_discrete_controller.mat');
        K  = data.K;
        u0 = data.u0;
        x0 = data.x0;
        ix = data.ix;
        iu = data.iu;
    end
    
    % State error
    dx = x - x0;
    
    % LQR control  (only selected states)
    du = -K * dx(ix);
    
    % Full control input
    u = u0;
    u(1:3) = u0(1:3) + du;   % only flap commands
end
